simulink model "untitled"  (R2019a)
settings: Solver=VariableStepAuto  StartTime=0.0  StopTime=120.0  RelTol=1e-3
values from neighbouring files (symbols this model uses):
  eps0 = [ -.5 ; -.5 ; .5 ]    [HW8.m]
  kd = I.*2*zeta*wn    [HW8.m]
  kp = 2.*I.*wn^2    [HW8.m]
undefined symbols (not defined in the file or in its folder): Td
settings Model: Creator=liamh  LastModifiedBy=liamh

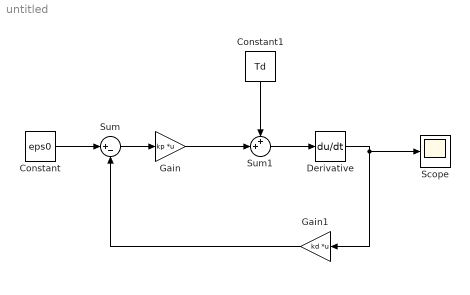
== system untitled ==
  Constant : Constant  Value=eps0  VectorParams1D=off
  Constant1 : Constant  Value=Td
  Derivative : Derivative
  Gain : Gain  Gain=kp  Multiplication=Matrix(K*u)
  Gain1 : Gain  Gain=kd  Multiplication=Matrix(K*u)
  Scope : Scope
  Sum : Sum  Inputs=|+-
  Sum1 : Sum  Inputs=++|
  wires:
  Constant/1 -> Sum/1
  Sum/1 -> Gain/1
  Gain/1 -> Sum1/2
  Constant1/1 -> Sum1/1
  Sum1/1 -> Derivative/1
  Derivative/1 -> Scope/1, Gain1/1
  Gain1/1 -> Sum/2
